simulink model "ANCfb"  (R2023b)
settings: Solver=ode3  StartTime=0.0  StopTime=10  RelTol=1e-3  EnableMultiTasking=on
libraries: matrix_library x52, dspadpt3 x31, raspberrypiAVlib x3
(part 2 of 2)

== system ANCfb/Audio Processing/Frame Breakdown/Subsystem1/Subsystem1 ==
  note: Anti-noise
  In1 : Inport
  In2 : Inport  Port=2
  Delay1 : Delay  DelayLength=1
  Estim. sec. path : DiscreteFir  Commented=through  Coefficients="[0.466  0.533  -0.257  -0.274  -0.231  -0.175]"
  Gain : Gain  Gain=-1
  LMS Update : dspadpt3/LMS Update  Method=Normalized LMS  Length=L  NumFilters=1  StepSizeSource=Property  StepSize=0.001  LeakageFactor=1.0  InitialConditions=0  AdaptiveFilterMode=Tapped delay-line FIR filter  EnableAdaptInput=off  EnableResetInput=off  SimulateUsing=Code generation
  LMS filter copy : DiscreteFir  CoefSource=Input port
      settings: InputPortMap=u0,u1
  y : Outport
  wires:
  Gain/1 -> y/1
  LMS filter copy/1 -> Gain/1
  Delay1/1 -> LMS filter copy/2
  LMS Update/1 -> Delay1/1
  Estim. sec. path/1 -> LMS Update/1
  In2/1 -> LMS Update/2
  In1/1 -> Estim. sec. path/1, LMS filter copy/1

== system ANCfb/Audio Processing/Frame Breakdown/Subsystem2/Subsystem2 ==
  note: Anti-noise
  In1 : Inport
  In2 : Inport  Port=2
  Delay1 : Delay  DelayLength=1
  Estim. sec. path : DiscreteFir  Commented=through  Coefficients="[0.466  0.533  -0.257  -0.274  -0.231  -0.175]"
  Gain : Gain  Gain=-1
  LMS Update : dspadpt3/LMS Update  Method=Normalized LMS  Length=L  NumFilters=1  StepSizeSource=Property  StepSize=0.001  LeakageFactor=1.0  InitialConditions=0  AdaptiveFilterMode=Tapped delay-line FIR filter  EnableAdaptInput=off  EnableResetInput=off  SimulateUsing=Code generation
  LMS filter copy : DiscreteFir  CoefSource=Input port
      settings: InputPortMap=u0,u1
  y : Outport
  wires:
  Gain/1 -> y/1
  LMS filter copy/1 -> Gain/1
  Delay1/1 -> LMS filter copy/2
  LMS Update/1 -> Delay1/1
  Estim. sec. path/1 -> LMS Update/1
  In2/1 -> LMS Update/2
  In1/1 -> Estim. sec. path/1, LMS filter copy/1

== system ANCfb/Audio Processing/Frame Breakdown/Subsystem3/Subsystem3 ==
  note: Anti-noise
  In1 : Inport
  In2 : Inport  Port=2
  Delay1 : Delay  DelayLength=1
  Estim. sec. path : DiscreteFir  Commented=through  Coefficients="[0.466  0.533  -0.257  -0.274  -0.231  -0.175]"
  Gain : Gain  Gain=-1
  LMS Update : dspadpt3/LMS Update  Method=Normalized LMS  Length=L  NumFilters=1  StepSizeSource=Property  StepSize=0.001  LeakageFactor=1.0  InitialConditions=0  AdaptiveFilterMode=Tapped delay-line FIR filter  EnableAdaptInput=off  EnableResetInput=off  SimulateUsing=Code generation
  LMS filter copy : DiscreteFir  CoefSource=Input port
      settings: InputPortMap=u0,u1
  y : Outport
  wires:
  Gain/1 -> y/1
  LMS filter copy/1 -> Gain/1
  Delay1/1 -> LMS filter copy/2
  LMS Update/1 -> Delay1/1
  Estim. sec. path/1 -> LMS Update/1
  In2/1 -> LMS Update/2
  In1/1 -> Estim. sec. path/1, LMS filter copy/1

== system ANCfb/Audio Processing/Frame Breakdown/Subsystem4/Subsystem4 ==
  note: Anti-noise
  In1 : Inport
  In2 : Inport  Port=2
  Delay1 : Delay  DelayLength=1
  Estim. sec. path : DiscreteFir  Commented=through  Coefficients="[0.466  0.533  -0.257  -0.274  -0.231  -0.175]"
  Gain : Gain  Gain=-1
  LMS Update : dspadpt3/LMS Update  Method=Normalized LMS  Length=L  NumFilters=1  StepSizeSource=Property  StepSize=0.001  LeakageFactor=1.0  InitialConditions=0  AdaptiveFilterMode=Tapped delay-line FIR filter  EnableAdaptInput=off  EnableResetInput=off  SimulateUsing=Code generation
  LMS filter copy : DiscreteFir  CoefSource=Input port
      settings: InputPortMap=u0,u1
  y : Outport
  wires:
  Gain/1 -> y/1
  LMS filter copy/1 -> Gain/1
  Delay1/1 -> LMS filter copy/2
  LMS Update/1 -> Delay1/1
  Estim. sec. path/1 -> LMS Update/1
  In2/1 -> LMS Update/2
  In1/1 -> Estim. sec. path/1, LMS filter copy/1

== system ANCfb/Audio Processing/Frame Breakdown/Subsystem5/Subsystem5 ==
  note: Anti-noise
  In1 : Inport
  In2 : Inport  Port=2
  Delay1 : Delay  DelayLength=1
  Estim. sec. path : DiscreteFir  Commented=through  Coefficients="[0.466  0.533  -0.257  -0.274  -0.231  -0.175]"
  Gain : Gain  Gain=-1
  LMS Update : dspadpt3/LMS Update  Method=Normalized LMS  Length=L  NumFilters=1  StepSizeSource=Property  StepSize=0.001  LeakageFactor=1.0  InitialConditions=0  AdaptiveFilterMode=Tapped delay-line FIR filter  EnableAdaptInput=off  EnableResetInput=off  SimulateUsing=Code generation
  LMS filter copy : DiscreteFir  CoefSource=Input port
      settings: InputPortMap=u0,u1
  y : Outport
  wires:
  Gain/1 -> y/1
  LMS filter copy/1 -> Gain/1
  Delay1/1 -> LMS filter copy/2
  LMS Update/1 -> Delay1/1
  Estim. sec. path/1 -> LMS Update/1
  In2/1 -> LMS Update/2
  In1/1 -> Estim. sec. path/1, LMS filter copy/1

== system ANCfb/Audio Processing/Frame Breakdown/Subsystem6/Subsystem6 ==
  note: Anti-noise
  In1 : Inport
  In2 : Inport  Port=2
  Delay1 : Delay  DelayLength=1
  Estim. sec. path : DiscreteFir  Commented=through  Coefficients="[0.466  0.533  -0.257  -0.274  -0.231  -0.175]"
  Gain : Gain  Gain=-1
  LMS Update : dspadpt3/LMS Update  Method=Normalized LMS  Length=L  NumFilters=1  StepSizeSource=Property  StepSize=0.001  LeakageFactor=1.0  InitialConditions=0  AdaptiveFilterMode=Tapped delay-line FIR filter  EnableAdaptInput=off  EnableResetInput=off  SimulateUsing=Code generation
  LMS filter copy : DiscreteFir  CoefSource=Input port
      settings: InputPortMap=u0,u1
  y : Outport
  wires:
  Gain/1 -> y/1
  LMS filter copy/1 -> Gain/1
  Delay1/1 -> LMS filter copy/2
  LMS Update/1 -> Delay1/1
  Estim. sec. path/1 -> LMS Update/1
  In2/1 -> LMS Update/2
  In1/1 -> Estim. sec. path/1, LMS filter copy/1

== system ANCfb/Audio Processing/Frame Breakdown/Subsystem7/Subsystem7 ==
  note: Anti-noise
  In1 : Inport
  In2 : Inport  Port=2
  Delay1 : Delay  DelayLength=1
  Estim. sec. path : DiscreteFir  Commented=through  Coefficients="[0.466  0.533  -0.257  -0.274  -0.231  -0.175]"
  Gain : Gain  Gain=-1
  LMS Update : dspadpt3/LMS Update  Method=Normalized LMS  Length=L  NumFilters=1  StepSizeSource=Property  StepSize=0.001  LeakageFactor=1.0  InitialConditions=0  AdaptiveFilterMode=Tapped delay-line FIR filter  EnableAdaptInput=off  EnableResetInput=off  SimulateUsing=Code generation
  LMS filter copy : DiscreteFir  CoefSource=Input port
      settings: InputPortMap=u0,u1
  y : Outport
  wires:
  Gain/1 -> y/1
  LMS filter copy/1 -> Gain/1
  Delay1/1 -> LMS filter copy/2
  LMS Update/1 -> Delay1/1
  Estim. sec. path/1 -> LMS Update/1
  In2/1 -> LMS Update/2
  In1/1 -> Estim. sec. path/1, LMS filter copy/1

== system ANCfb/Audio Processing/Frame Breakdown/Subsystem8/Subsystem8 ==
  note: Anti-noise
  In1 : Inport
  In2 : Inport  Port=2
  Delay1 : Delay  DelayLength=1
  Estim. sec. path : DiscreteFir  Commented=through  Coefficients="[0.466  0.533  -0.257  -0.274  -0.231  -0.175]"
  Gain : Gain  Gain=-1
  LMS Update : dspadpt3/LMS Update  Method=Normalized LMS  Length=L  NumFilters=1  StepSizeSource=Property  StepSize=0.001  LeakageFactor=1.0  InitialConditions=0  AdaptiveFilterMode=Tapped delay-line FIR filter  EnableAdaptInput=off  EnableResetInput=off  SimulateUsing=Code generation
  LMS filter copy : DiscreteFir  CoefSource=Input port
      settings: InputPortMap=u0,u1
  y : Outport
  wires:
  Gain/1 -> y/1
  LMS filter copy/1 -> Gain/1
  Delay1/1 -> LMS filter copy/2
  LMS Update/1 -> Delay1/1
  Estim. sec. path/1 -> LMS Update/1
  In2/1 -> LMS Update/2
  In1/1 -> Estim. sec. path/1, LMS filter copy/1

== system ANCfb/Audio Processing/Frame Breakdown/Subsystem9/Subsystem9 ==
  note: Anti-noise
  In1 : Inport
  In2 : Inport  Port=2
  Delay1 : Delay  DelayLength=1
  Estim. sec. path : DiscreteFir  Commented=through  Coefficients="[0.466  0.533  -0.257  -0.274  -0.231  -0.175]"
  Gain : Gain  Gain=-1
  LMS Update : dspadpt3/LMS Update  Method=Normalized LMS  Length=L  NumFilters=1  StepSizeSource=Property  StepSize=0.001  LeakageFactor=1.0  InitialConditions=0  AdaptiveFilterMode=Tapped delay-line FIR filter  EnableAdaptInput=off  EnableResetInput=off  SimulateUsing=Code generation
  LMS filter copy : DiscreteFir  CoefSource=Input port
      settings: InputPortMap=u0,u1
  y : Outport
  wires:
  Gain/1 -> y/1
  LMS filter copy/1 -> Gain/1
  Delay1/1 -> LMS filter copy/2
  LMS Update/1 -> Delay1/1
  Estim. sec. path/1 -> LMS Update/1
  In2/1 -> LMS Update/2
  In1/1 -> Estim. sec. path/1, LMS filter copy/1
